simulink model "rl_final"  (R2017a)
settings: Solver=VariableStepAuto  StartTime=0.0  StopTime=inf  RelTol=1e-3
libraries: vrlib x3, sharedtransform x1
settings Model: Creator=Jarvis  LastModifiedBy=Jarvis

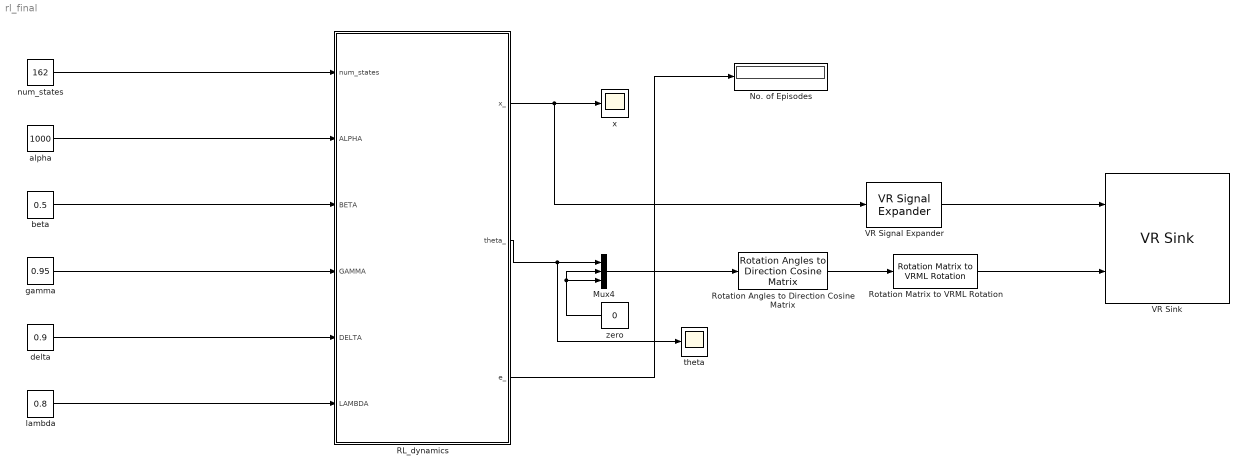
== system rl_final ==
  Mux4 : Mux  Inputs=3
  No. of Episodes : Display
  RL_dynamics : MATLAB Function  TreatAsAtomicUnit=on
  Rotation Angles to Direction Cosine Matrix : sharedtransform/Rotation Angles to Direction Cosine Matrix  rotationOrder=ZYX
      settings: SourceProductBaseCode=AE
  Rotation Matrix to VRML Rotation : vrlib/Utilities/Rotation Matrix to VRML Rotation  maxzero=1e-12
      settings: SourceProductName=Simulink 3D Animation  SourceProductBaseCode=VR
  VR Signal Expander : vrlib/VR Signal Expander  outwidth=3  outidx=[1]
      settings: SourceProductName=Simulink 3D Animation  SourceProductBaseCode=VR
  VR Sink : vrlib/VR Sink  InstantiateOnLoad=on  SampleTime=0.01  ViewEnable=on  RemoteChange=off  RemoteView=off  FieldsWritten=Cart.translation.3.1.1.double#Pendulum.rotation.4.1.1.double  WorldFileName=Inverted_Pendulum.wrl  AutoView=off  VideoDimensions=[]  AllowVariableSize=off
      settings: SourceProductBaseCode=VR
  alpha : Constant  Value=1000
  beta : Constant  Value=0.5
  delta : Constant  Value=0.9
  gamma : Constant  Value=0.95
  lambda : Constant  Value=0.8
  num_states : Constant  Value=162
  theta : Scope
  x : Scope
  zero : Constant  Value=0
  wires:
  num_states/1 -> RL_dynamics/1(num_states)
  alpha/1 -> RL_dynamics/2(ALPHA)
  beta/1 -> RL_dynamics/3(BETA)
  gamma/1 -> RL_dynamics/4(GAMMA)
  delta/1 -> RL_dynamics/5(DELTA)
  lambda/1 -> RL_dynamics/6(LAMBDA)
  Rotation Angles to Direction Cosine Matrix/1 -> Rotation Matrix to VRML Rotation/1
  Mux4/1 -> Rotation Angles to Direction Cosine Matrix/1
  zero/1 -> Mux4/2, Mux4/3
  VR Signal Expander/1 -> VR Sink/1
  RL_dynamics/1(x_) -> VR Signal Expander/1, x/1
  Rotation Matrix to VRML Rotation/1 -> VR Sink/2
  RL_dynamics/2(theta_) -> theta/1, Mux4/1
  RL_dynamics/3(e_) -> No. of Episodes/1

== matlab function rl_final/RL_dynamics ==
  data: x_ output; theta_ output; num_states input; ALPHA input; BETA input; GAMMA input; DELTA input; LAMBDA input; e_ output
function [x_, theta_, e_] = fcn(num_states, ALPHA, BETA, GAMMA, DELTA, LAMBDA)

    persistent w;
    persistent fail_flag;
    persistent v;
    persistent xbar;
    persistent e;
    persistent trial;
    persistent episode;
    persistent x;
    persistent theta;
    persistent x_dot;
    persistent theta_dot;
    persistent index;
    persistent p_t_1;
    persistent y;
    persistent r;
    persistent p;
    persistent rcap;
    
    if isempty(fail_flag)
        fail_flag = 0;
    end
    if isempty(r)
        r = 0;
    end
    if isempty(p)
        p = 0;
    end
    if isempty(rcap)
        rcap = 0;
    end
    if isempty(y)
        y = 0;
    end
    if isempty(p_t_1)
        p_t_1 = 0;
    end
    if isempty(index)
        index = 0;
    end
    if isempty(x)
        x = 0;
    end
    if isempty(theta)
        theta = 0;
    end
    if isempty(x_dot)
        x_dot = 0;
    end
    if isempty(theta_dot)
        theta_dot = 0;
    end
    if isempty(trial)
        trial = 0;
    end
    if isempty(episode)
        episode = 0;
    end
    if isempty(w)
        w = zeros(162, 1);      %Weights for ASE
    end
    if isempty(v)
        v = zeros(162, 1);      %Weights for ACE
    end
    if isempty(xbar)
        xbar = zeros(162, 1);   %Decay vector for ACE
    end
    if isempty(e)
        e = zeros(162, 1);      %Decay vector for ASE
    end
    j = 0;
    %Initialise states to zero.
    % x = 0;
    % x_dot = 0;
    % theta = 0;
    % theta_dot = 0;

    %Get the index of the state vector from the decoder.
    index = decoder(x, x_dot, theta, theta_dot);

    %Initially, increment the episode to 1.
    %Generate noise and use sigmoid activation function, and then generate
    %the signum function value for y i.e the action y = [0,1].  
    noise = rand() * 10e-4;
    y = double(noise < sigmoid(w(index + 1)));

    %Apply the force to the system and capture its new states.
    [x, x_dot, theta, theta_dot] = dynamics(y, x, x_dot, theta, theta_dot);

    %increment index as matlab indexing is from 1.
    e(index+1) = e(index+1) + (1-DELTA) * (y - 0.5);    %Update traces from 't-1' to 't'
    xbar(index + 1) = xbar(index + 1) + (1-LAMBDA);

    %Store the 't-1' value of v vector to compute the prediction equation.
    p_t_1 = v(index + 1);

    %{
    disp("==========================");
    fprintf("x = %d x_dot = %d theta = %d theta_dot = %d \n", x, x_dot, theta, theta_dot);
    %}

    %After applying force, get the state vector from the decoder.
    index = decoder(x, x_dot, theta, theta_dot);

    %Check if pole has fallen.
    if(index < 0)
        %Pole has fallen.
        fail_flag = 1;              %Turn on the fail flag so that we can reset the states to [0 0 0 0]'
        episode = episode + 1;      %Increment the number of episodes
        %fprintf("Episode %d occured with %d trials.\n", episode, trial);
        trial = 0;                  %Reset the trial to zero.

        %Reset all the state variables.
        x = 0;
        x_dot = 0;
        theta = 0;
        theta_dot = 0;

        %Read the new index after resetting.
        index = decoder(x, x_dot, theta, theta_dot);

        %Make the reward -1, and reset the prediction to zero.
        r = -1;
        p = 0;
    else
        %Pole has not yet fallen. keep fail flag nonzero so that
        %unnecessary reset doesnt occur. reward is set to zero and the
        %prediction value is updated.
        fail_flag = 0;
        r = 0;
        p = v(index + 1);
    end

    %Compute the reward for the ASE.
    rcap = r + GAMMA * p - p_t_1;

    %Update the weights for ASE and ACE. Weights for ACE are constrained to
    %be greater than -1, so that the equations converge.
    w = w + ALPHA * rcap * e;
    v = v + BETA * rcap * xbar;
    for j = 1:num_states
        if(v(j) < -1)
            v(j) = v(j);
        end
    end

    %If fail flag is zero, reset the decay functions.
    if(fail_flag)
        e = zeros(162, 1);
        xbar = zeros(162, 1);
    else
        %Update the decay functions from 't-1' to current 't'
        e = e * DELTA;
        xbar = xbar * LAMBDA;
    end
    %Increment the trials.
    trial = trial + 1;
    x_ = x;
    theta_ = theta;
    e_ = episode;
end

function[x_, x_dot_, theta_, theta_dot_] = dynamics(action, x, x_dot, theta, theta_dot)
    g = 9.81;
    M = 1.0;
    m = 0.1;
    Mm = m + M;
    l = 0.5;
    ml = m * l;
    t = 0.02;
    
    if action > 0
        f = 10;
    else
        f = -10;
    end
    
    costheta = cos(theta);
    sintheta = sin(theta);
    
    numerator_2 = (f + ml * theta_dot * theta_dot * sintheta)/Mm;
    thetaacc = (g * sintheta - costheta*numerator_2)/(l * ((4/3) - m * costheta * costheta / Mm));
    xacc = numerator_2 - ml * thetaacc * costheta / Mm;
    
    x_ = x + t * x_dot;
    x_dot_ = x_dot + t * xacc;
    theta_ = theta + t * theta_dot;
    theta_dot_ = theta_dot + t * thetaacc;
    
end

function s_ = sigmoid(s)
    s_ = 1/(1 + exp(-max(-50, min(s, 50))));
end


function index = decoder(x, x_dot, theta, theta_dot)
    %fprintf("x = %d x_dot = %d theta = %d theta_dot = %d \n", x, x_dot, theta, theta_dot);
    %disp("==========================");
    index = 0;
    theta = (180/pi)*theta;
    theta_dot = (180/pi)*theta_dot;
    if(x < -2.4 || x > 2.4|| theta < -12 || theta > 12)
        index = -1;
        return;
    end
    
    if(x < -0.8)    
        index = 0;
    elseif(x < 0.8)     
        index = 1;
    else
        index = 2;
    end
    
    if(x_dot < -0.5)
        %do nothing
    elseif(x_dot < 0.5)     
        index = index + 3;
    else
        index = index + 6;
    end
    
    if (theta < -6) 	
        %do nothing
    elseif (theta < -1) 
        index = index + 9;
    elseif (theta < 0)  
        index = index + 18;
    elseif (theta < 1)  
        index = index + 27;
    elseif (theta < 6)  
        index = index + 36;
    else
        index = index + 45;
    end
    
    if (theta_dot < -50) 	 
        %do nothing
    elseif (theta_dot < 50)  
        index = index + 54;
    else
        index = index + 108;
    end
end
